simulink model "Closed_Loop"  (R2018b)
settings: Solver=VariableStepAuto  StartTime=0.0  StopTime=t_f  RelTol=1e-3
values from neighbouring files (symbols this model uses):
  A = [ A_1_1 A_1_2 0 A_1_4 ... (first row only)    [Master.m]
  B = [B_1 ... (first row only)    [Master.m]
  K = place(A,B,p)    [Master.m]
settings Model: Creator=Cam  LastModifiedBy=Cam

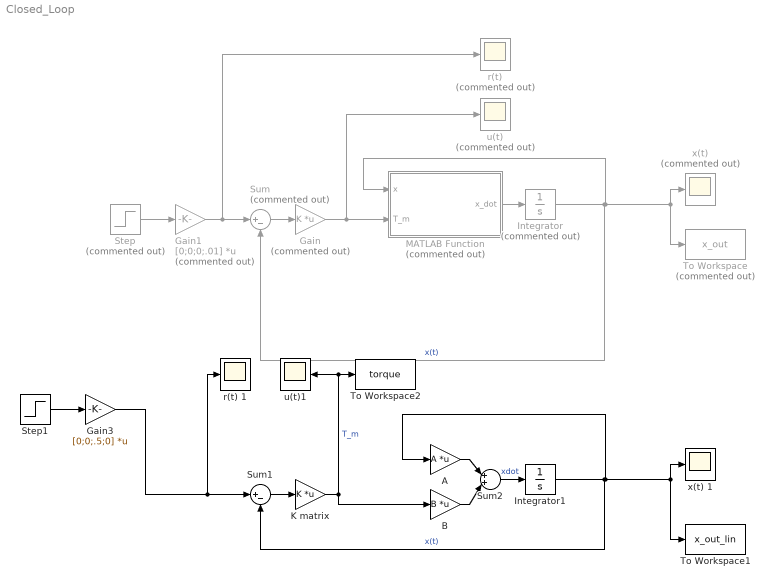
== system Closed_Loop ==
  A : Gain  Gain=A  Multiplication=Matrix(K*u)
  B : Gain  Gain=B  Multiplication=Matrix(K*u)
  Gain : Gain  Commented=on  Gain=K  Multiplication=Matrix(K*u)
  Gain1 : Gain  Commented=on  Gain=[0;0;0;.01]  Multiplication=Matrix(K*u)
  Gain3 : Gain  Gain=[0;0;.5;0]  Multiplication=Matrix(K*u)
  Integrator : Integrator  Commented=on  InitialCondition=[0;0;0;.1]
  Integrator1 : Integrator  InitialCondition=[0;0;0;.1]
  K matrix : Gain  Gain=K  Multiplication=Matrix(K*u)
  MATLAB Function : MATLAB Function  Commented=on  TreatAsAtomicUnit=on
  Step : Step  Commented=on  After=0  SampleTime=0
  Step1 : Step  Time=5  SampleTime=0
  Sum : Sum  Commented=on  Inputs=|+-
  Sum1 : Sum  Inputs=|+-
  Sum2 : Sum  Inputs=|++|
  To Workspace : ToWorkspace  Commented=on  VariableName=x_out  SampleTime=-1
  To Workspace1 : ToWorkspace  VariableName=x_out_lin  SampleTime=-1
  To Workspace2 : ToWorkspace  VariableName=torque  SampleTime=-1
  "r(t) " : Scope  Commented=on
  r(t) 1 : Scope
  u(t) : Scope  Commented=on
  u(t)1 : Scope
  "x(t) " : Scope  Commented=on
  x(t) 1 : Scope
  wires:
  MATLAB Function/1(x_dot) -> Integrator/1
  Integrator/1 -> To Workspace/1, "x(t) "/1, MATLAB Function/1(x), Sum/2  "x(t)"
  Step/1 -> Gain1/1
  Sum/1 -> Gain/1
  Gain/1 -> MATLAB Function/2(T_m), u(t)/1
  Gain1/1 -> "r(t) "/1, Sum/1
  Sum1/1 -> K matrix/1
  Gain3/1 -> Sum1/1, r(t) 1/1
  K matrix/1 -> B/1, To Workspace2/1, u(t)1/1  "T_m"
  Step1/1 -> Gain3/1
  Integrator1/1 -> A/1, To Workspace1/1, x(t) 1/1, Sum1/2  "x(t)"
  Sum2/1 -> Integrator1/1  "xdot"
  B/1 -> Sum2/2
  A/1 -> Sum2/1

== matlab function Closed_Loop/MATLAB Function ==
  data: x input; x_dot output; T_m input
function x_dot  = botEOM(x, T_m)

%% Variables
g = 32.174;   %gravity
weight_1=1.1/16;    %weight of wheel, lbf
weight_2=1.63-2*weight_1;       %weight of body, lbf
m_1 = weight_1/g; %mass of wheel, slug
m_2 = weight_2/g; %mass of body
r_1 = 2.55/2; %radius of wheel
r_2 = 1.028; %distance from center of wheel to c.g. of body
I_1 = m_1*r_1^2; %moment of inertia of wheel slug*in^2
I_2 = 1; %moment of inertia of body

m_eff =  m_1 + m_2 + (I_1/r_1^2); %effective mass
I_eff = m_2*r_2^2 + I_2; %effective moment of inertia
b_1 = 0; %damping coefficient from rolling resistance due to translation of x
b_2 = 0; %damping coefficient relative from rolling between wheels to body (theta 2-theta1)

%% matrices
A1 = [m_eff -m_2*r_2*cos(x(4)) 0 0
     -m_2*r_2*cos(x(4)) I_eff 0 0
      0 0 1 0
      0 0 0 1];
A2 = [-T_m/r_1 - (b_2/r_1^2)*x(1) - (b_2/r_1)*x(2) - b_1*x(1) - m_2*r_2*x(2)^2*sin(x(4))
    T_m - (b_2/r_1)*x(1) - b_2*x(2) + m_2*r_2*g*sin(x(4))
    x(1)
    x(2)];

x_dot = A1\A2;
